simulink model "c8mchuasim"  (R2019b)
settings: Solver=ode15s  StartTime=0.0  StopTime=500  FixedStep=0.001  RelTol=1e-9  EnableMultiTasking=on
PreLoadFcn:
  | alpha=[0.93,0.99,0.92]; x0=[0.2; -0.1; 0.1];
  | a=10.725; b=10.593; c=0.268; m0=-1.1726; m1=-0.7872;
  | ww=[1e-4 1e3]; N=13;
libraries: cstblocks x3
settings Model: Creator=toshiba  LastModifiedBy=xuedi
settings DataIOCC: MaxDataPoints=10000  SaveFormat=Array  SignalLoggingSaveFormat=ModelDataLogs  ReturnWorkspaceOutputs=off
settings OptimizationCC: ExpressionDepthLimit=2147483647  LifeSpan=inf
settings DebuggingCC: UnderspecifiedInitializationDetection=Classic  MergeDetectMultiDrivingBlocksExec=none  FcnCallInpInsideContextMsg=warning  StateNameClashWarn=warning  SFUnexpectedBacktrackingDiag=warning  SFNoUnconditionalDefaultTransitionDiag=warning  SFExecutionAtInitializationDiag=none  ArithmeticOperatorsInVariantConditions=warning
settings HardwareCC: ProdBitPerPointer=32  ProdBitPerSizeT=32  ProdBitPerPtrDiffT=32  ProdLargestAtomicFloat=None  ProdIntDivRoundTo=Undefined  ProdEndianess=Unspecified  ProdWordSize=32  ProdHWDeviceType=32-bit Generic
settings ModelReferenceCC: PropagateSignalLabelsOutOfModel=off
settings SFSimCC: SimUseLocalCustomCode=off  CustomCodeUndefinedFunction=UseInterfaceOnly
settings RTWCC: RTWUseLocalCustomCode=off
settings CodeAppCC: StateflowObjectComments=on
settings GRTTargetCC: TargetLangStandard=C89/C90 (ANSI)  CombineOutputUpdateFcns=off  GRTInterface=on
settings ConfigComp: CovMetricSettings=dw  CovSaveCumulativeToWorkspaceVar=on  CovSaveSingleToWorkspaceVar=on  CovExternalEMLEnable=off

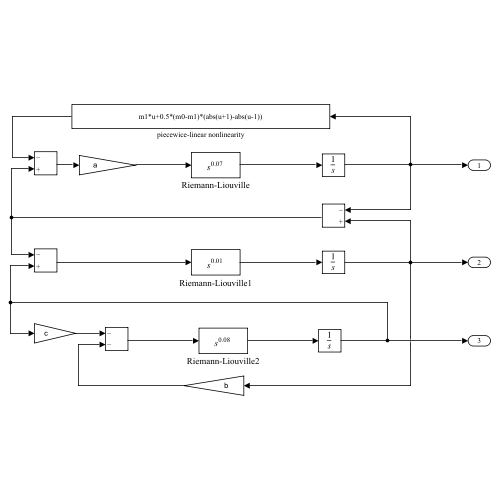
[thumbnail: Simulink's stored preview of the top-level diagram]
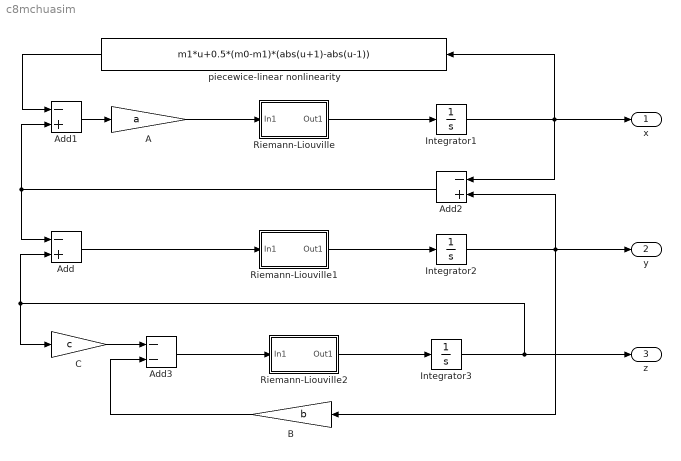
== system c8mchuasim ==
  A : Gain  Gain=a
  Add : Sum  Inputs=-+
  Add1 : Sum  Inputs=-+
  Add2 : Sum  Inputs=-+
  Add3 : Sum  Inputs=--
  B : Gain  Gain=b
  C : Gain  Gain=c
  Integrator1 : Integrator  InitialCondition=0.2
  Integrator2 : Integrator  InitialCondition=-0.1
  Integrator3 : Integrator  InitialCondition=0.1
  Riemann-Liouville : Subsystem  mask{gam=1-alpha(1), ww=ww, n=N, kF1=off, kF=Oustaloup filter}
      mask prompts: gam "Derivative order gamma"; ww "Frequency range [wb,wh]"; n "Apprixmation order"; kF1 "Is a low-pass filter required?"; kF "Filter type"
      mask init:
      | wb=ww(1); wh=ww(2); 
      |    if isnumeric(gam), str=['{\its}^{' num2str(gam) '}']; 
      |    else, str='{\its}^{\gamma}'; end
      |    switch kF
      |       case 1, G=ousta_fod(gam,n,wb,wh);
      |       case 2, G=new_fod(gam,n,wb,wh); 
      |       case 3, G=matsuda_fod(gam,n,wb,wh); 
      |       case 4, G=srid_fod(gam,0.01,n);
      |    end
      |    T=1e-6/wh; if kF1==1, G=G*tf(1,[T 1]); end
      mask TypeOptions kF: Oustaloup filter | Modified Oustaloup filter | Matsuda-Fujii filter | Discrete step invariant filter
      mask Display: disp(str,'texmode','on')
  Riemann-Liouville1 : Subsystem  mask{gam=1-alpha(2), ww=ww, n=N, kF1=off, kF=Oustaloup filter}
      mask prompts: gam "Derivative order gamma"; ww "Frequency range [wb,wh]"; n "Apprixmation order"; kF1 "Is a low-pass filter required?"; kF "Filter type"
      mask init: same as c8mchuasim/Riemann-Liouville
      mask TypeOptions kF: Oustaloup filter | Modified Oustaloup filter | Matsuda-Fujii filter | Discrete step invariant filter
      mask Display: disp(str,'texmode','on')
  Riemann-Liouville2 : Subsystem  mask{gam=1-alpha(3), ww=ww, n=N, kF1=off, kF=Oustaloup filter}
      mask prompts: gam "Derivative order gamma"; ww "Frequency range [wb,wh]"; n "Apprixmation order"; kF1 "Is a low-pass filter required?"; kF "Filter type"
      mask init: same as c8mchuasim/Riemann-Liouville
      mask TypeOptions kF: Oustaloup filter | Modified Oustaloup filter | Matsuda-Fujii filter | Discrete step invariant filter
      mask Display: disp(str,'texmode','on')
  piecewice-linear nonlinearity : Fcn  Expr=m1*u+0.5*(m0-m1)*(abs(u+1)-abs(u-1))
  x : Outport
  y : Outport  Port=2
  z : Outport  Port=3
  wires:
  Add1/1 -> A/1
  Integrator1/1 -> x/1, Add2/1, piecewice-linear nonlinearity/1
  piecewice-linear nonlinearity/1 -> Add1/1
  Add2/1 -> Add/1, Add1/2
  Integrator2/1 -> y/1, B/1, Add2/2
  Integrator3/1 -> z/1, C/1, Add/2
  C/1 -> Add3/1
  B/1 -> Add3/2
  A/1 -> Riemann-Liouville/1(In1)
  Add/1 -> Riemann-Liouville1/1(In1)
  Add3/1 -> Riemann-Liouville2/1(In1)
  Riemann-Liouville/1(Out1) -> Integrator1/1
  Riemann-Liouville1/1(Out1) -> Integrator2/1
  Riemann-Liouville2/1(Out1) -> Integrator3/1

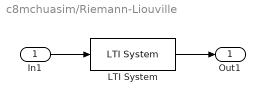
== system c8mchuasim/Riemann-Liouville ==
  In1 : Inport
  LTI System : cstblocks/LTI System  sys=G  IC=[]
  Out1 : Outport
  wires:
  In1/1 -> LTI System/1
  LTI System/1 -> Out1/1

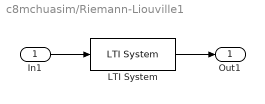
== system c8mchuasim/Riemann-Liouville1 ==
  In1 : Inport
  LTI System : cstblocks/LTI System  sys=G  IC=[]
  Out1 : Outport
  wires:
  LTI System/1 -> Out1/1
  In1/1 -> LTI System/1

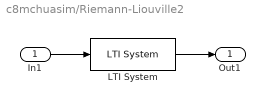
== system c8mchuasim/Riemann-Liouville2 ==
  In1 : Inport
  LTI System : cstblocks/LTI System  sys=G  IC=[]
  Out1 : Outport
  wires:
  In1/1 -> LTI System/1
  LTI System/1 -> Out1/1
